simulink model "Copy_of_calibration_pumps"  (R2026a)
settings: Solver=VariableStepAuto  StopTime=inf
StopFcn:
  | Q = out.Q;Q = out.Q;
  | 
  | folder = 'calibration_data';
  | 
  | if ~exist(folder, 'dir')
  |     mkdir(folder);
  | end
  | 
  | baseName = 'pump_calibration';
  | fileName = fullfile(folder, baseName + ".mat");
  | 
  | n = 2;
  | 
  | while exist(fileName, 'file')
  |     fileName = fullfile(folder, baseName + "_" + n + ".mat");
  |     n = n + 1;
  | end
  | 
  | save(fileName, 'Q');
  | 
  | fprintf('Calibration saved to: %s\n', fileName);
values from neighbouring files (symbols this model uses):
  coefficients = [20.111978783 20.2762923351 20.4770477048]    [sensor_calibration.mat]
settings Model: Creator=user  LastModifiedBy=user

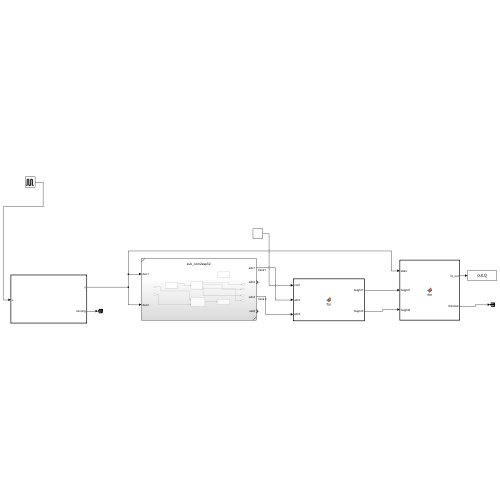
[thumbnail: Simulink's stored preview of the top-level diagram]
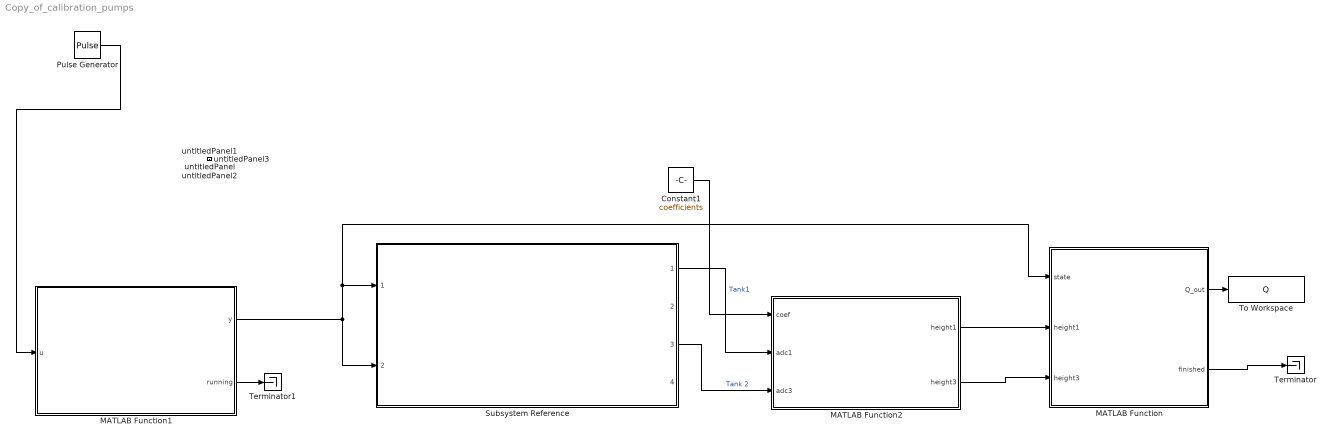
== system Copy_of_calibration_pumps ==
  Constant1 : Constant  Value=coefficients
  MATLAB Function : MATLAB Function  TreatAsAtomicUnit=on
  MATLAB Function1 : MATLAB Function  TreatAsAtomicUnit=on
  MATLAB Function2 : MATLAB Function  TreatAsAtomicUnit=on
  Pulse Generator : DiscretePulseGenerator  PulseType=Time based  Period=12  PulseWidth=20
  Subsystem Reference : Subsystem  ReferencedSubsystem=sub_com2esp32
  Terminator : Terminator
  Terminator1 : Terminator
  To Workspace : ToWorkspace  VariableName=Q  SampleTime=-1
      settings: MaxDataPoints=1
  untitledPanel : Subsystem  Tag=HiddenForWebPanel  IsWebBlockPanel=on
  untitledPanel1 : Subsystem  Tag=HiddenForWebPanel  IsWebBlockPanel=on
  untitledPanel2 : Subsystem  Tag=HiddenForWebPanel  IsWebBlockPanel=on
  untitledPanel3 : Subsystem  Tag=HiddenForWebPanel  IsWebBlockPanel=on
  wires:
  MATLAB Function/1(Q_out) -> To Workspace/1
  MATLAB Function/2(finished) -> Terminator/1
  MATLAB Function1/1(y) -> MATLAB Function/1(state), Subsystem Reference/1, Subsystem Reference/2
  MATLAB Function1/2(running) -> Terminator1/1
  Pulse Generator/1 -> MATLAB Function1/1(u)
  Subsystem Reference/1 -> MATLAB Function2/2(adc1)  "Tank1"
  Subsystem Reference/3 -> MATLAB Function2/3(adc3)  "Tank 2"
  Constant1/1 -> MATLAB Function2/1(coef)
  MATLAB Function2/1(height1) -> MATLAB Function/2(height1)
  MATLAB Function2/2(height3) -> MATLAB Function/3(height3)

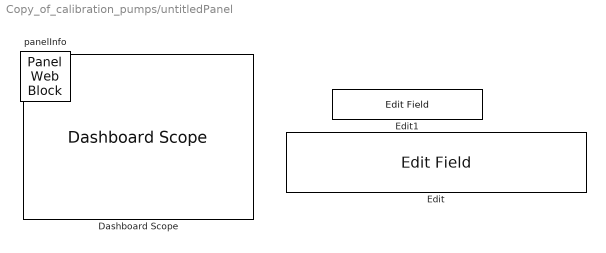
== system Copy_of_calibration_pumps/untitledPanel ==
  Dashboard Scope : DashboardScope  Tag=HiddenForWebPanel  PanelInfo="{\"height\":195,\"left\":22,\"panelId\":\"panelId-0a8f6d05-5e0e-4052-8464-4cdde78ccbfe\",\"top\":22,\"type\":\"panelChild\",\"version\":\"2019b\",\"width\":271,\"zIndex\":1500002}"  FontColor=[0.0, 0.0, 0.0]
  Edit : EditField  Tag=HiddenForWebPanel  PanelInfo="{\"height\":25,\"left\":322,\"panelId\":\"panelId-0a8f6d05-5e0e-4052-8464-4cdde78ccbfe\",\"top\":100,\"type\":\"panelChild\",\"version\":\"2019b\",\"width\":181,\"zIndex\":1500006}"  LabelPosition=Hide  ShowInitialText=on  Alignment=Center
  Edit1 : EditField  Tag=HiddenForWebPanel  PanelInfo="{\"height\":30,\"left\":327,\"panelId\":\"panelId-0a8f6d05-5e0e-4052-8464-4cdde78ccbfe\",\"top\":53,\"type\":\"panelChild\",\"version\":\"2019b\",\"width\":150,\"zIndex\":1500004}"  LabelPosition=Hide  ShowInitialText=on  Alignment=Center
  panelInfo : PanelWebBlock  Tag=HiddenForWebPanel  PanelInfo="{\"compacted\":false,\"height\":362,\"isActiveTab\":false,\"left\":183,\"name\":\"Panel\",\"panelId\":\"panelId-0a8f6d05-5e0e-4052-8464-4cdde78ccbfe\",\"popoutData\":{\"height\":495,\"left\":546,\"maximized\":false,\"top\":827,\"width\":618},\"popoutMode\":\"windowHidden\",\"tabIndex\":0,\"tabbedSetId\":\"tabbedSet4972758365\",\"top\":737,\"type\":\"panel\",\"version\":\"2019b\",\"visible\":false,\"width\":602,\"zIndex\":1500002}"  PanelSnapshot=<binary blob, 20028 chars, not shown>

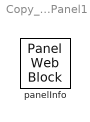
== system Copy_of_calibration_pumps/untitledPanel1 ==
  panelInfo : PanelWebBlock  Tag=HiddenForWebPanel  PanelInfo="{\"compacted\":false,\"height\":362,\"isActiveTab\":true,\"left\":183,\"name\":\"Panel1\",\"panelId\":\"panelId-b2ee2f41-7720-49f1-b51a-3062c351f597\",\"popoutData\":{\"height\":495,\"left\":546,\"maximized\":false,\"top\":827,\"width\":618},\"popoutMode\":\"windowHidden\",\"tabIndex\":1,\"tabbedSetId\":\"tabbedSet4972758365\",\"top\":737,\"type\":\"panel\",\"version\":\"2019b\",\"visible\":true,\"width\":602,\"zIndex\":1500004}"

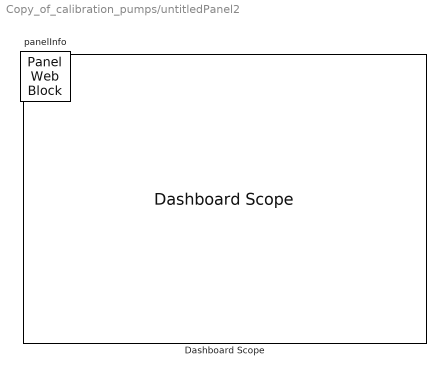
== system Copy_of_calibration_pumps/untitledPanel2 ==
  Dashboard Scope : DashboardScope  Tag=HiddenForWebPanel  PanelInfo="{\"height\":289,\"left\":18,\"panelId\":\"panelId-8ba459e9-7eb9-43d1-9a8b-2b7bff5a2d5c\",\"top\":18,\"type\":\"panelChild\",\"version\":\"2019b\",\"width\":403,\"zIndex\":1500002}"  FontColor=[0.0, 0.0, 0.0]
  panelInfo : PanelWebBlock  Tag=HiddenForWebPanel  PanelInfo="{\"compacted\":false,\"height\":329,\"isActiveTab\":true,\"left\":1320,\"name\":\"Panel2\",\"panelId\":\"panelId-8ba459e9-7eb9-43d1-9a8b-2b7bff5a2d5c\",\"popoutData\":{\"height\":440,\"left\":1683,\"maximized\":false,\"top\":822,\"width\":459},\"popoutMode\":\"windowHidden\",\"tabIndex\":0,\"tabbedSetId\":\"tabbedSet1724704130\",\"top\":710,\"type\":\"panel\",\"version\":\"2019b\",\"visible\":true,\"width\":443,\"zIndex\":1500006}"  PanelSnapshot=<binary blob, 75208 chars, not shown>

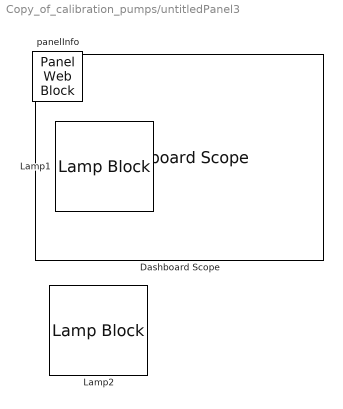
== system Copy_of_calibration_pumps/untitledPanel3 ==
  Dashboard Scope : DashboardScope  Tag=HiddenForWebPanel  PanelInfo="{\"height\":364,\"left\":211,\"panelId\":\"panelId-037cc253-1a0e-430c-bfc3-d197bdfa8fb6\",\"top\":20,\"type\":\"panelChild\",\"version\":\"2019b\",\"width\":531,\"zIndex\":1500002}"  Ymin=0  FontColor=[0.0, 0.0, 0.0]
  Lamp1 : LampBlock  Tag=HiddenForWebPanel  PanelInfo="{\"height\":82,\"left\":28,\"panelId\":\"panelId-037cc253-1a0e-430c-bfc3-d197bdfa8fb6\",\"top\":79,\"type\":\"panelChild\",\"version\":\"2019b\",\"width\":89,\"zIndex\":1500004}"  LabelPosition=Hide  DefaultColor=[192.0, 192.0, 192.0]
  Lamp2 : LampBlock  Tag=HiddenForWebPanel  PanelInfo="{\"height\":82,\"left\":29,\"panelId\":\"panelId-037cc253-1a0e-430c-bfc3-d197bdfa8fb6\",\"top\":226,\"type\":\"panelChild\",\"version\":\"2019b\",\"width\":89,\"zIndex\":1500006}"  LabelPosition=Hide  DefaultColor=[192.0, 192.0, 192.0]
  panelInfo : PanelWebBlock  Tag=HiddenForWebPanel  PanelInfo="{\"compacted\":false,\"height\":411,\"isActiveTab\":true,\"labels\":{\"label0415151059\":{\"deleted\":false,\"left\":29,\"settings\":{\"backgroundColor\":\"rgba(0, 0, 0, 0)\",\"bold\":true,\"font\":\"Arial\",\"fontColor\":\"black\",\"fontSize\":1.09,\"italicized\":false,\"underlined\":false},\"text\":\"Pump\",\"top\":54},\"label6487320007\":{\"deleted\":false,\"left\":27,\"settings\":{\"backgroundColor\":\"rgba(0, 0, 0, 0)\",\"bold\":true,\"font\":\"Arial\",\"fontColor\":\"black\",\"fontSize\":1,\"italicized\":false,\"underlined\":false},\"text\":\"Calibration finished\",\"top\":201}},\"left\":1544,\"name\":\"Panel3\",\"panelId\":\"panelId-037cc253-1a0e-430c-bfc3-d197bdfa8fb6\",\"tabIndex\":0,\"tabbedSetId\":\"tabbedSet3591606152\",\"top\":209,\"type\":\"panel\",\"version\":\"2019b\",\"visible\":true,\"width\":760,\"zIndex\":1500008}"  PanelSnapshot=<binary blob, 44244 chars, not shown>

== matlab function Copy_of_calibration_pumps/MATLAB Function ==
  data: state input; Q_out output; finished output; height1 input; height3 input
function [Q_out, finished] = fcn(state, height1, height3)

persistent sensor_low prev_state Q counter

if isempty(sensor_low)

    sensor_low = zeros(2,1);
    prev_state = 255;
    counter = 0;

    Q = zeros(2,9);

end

A = 154;
dt = 12 * 0.8;

finished = 0;

sensor_now = [height1; height3] * A;

if state ~= 255 && prev_state == 255

    counter = counter + 1;

    if counter <= 8
        sensor_low = sensor_now;
    end

end

if state == 255 && prev_state ~= 255

    if counter >= 1 && counter <= 8

        sensor_high = sensor_now;

        Q(:,counter+1) = ...
            (sensor_high - sensor_low) / dt;

    end

end

if counter >= 8 && state == 255
    finished = 1;
end

prev_state = state;

Q_out = Q;

end

== matlab function Copy_of_calibration_pumps/MATLAB Function1 ==
  data: u input; y output; running output
function [y,running] = fcn(u)
persistent counter2 prev_u

if isempty(counter2) && isempty(prev_u)
    counter2 =0; 
    prev_u =0; 
end
running = 1;

if u ==1 && prev_u ==0
    counter2 = counter2 +1;
end
if u ==0
    s = 0.125 * counter2; 
    if s <= 1
        y = 255 * (1-s);
        running =0;
    else 
        y = 255; 
    end
else
    y = 255; 
end

prev_u = u;

== matlab function Copy_of_calibration_pumps/MATLAB Function2 ==
  data: coef input; height1 output; adc1 input; adc3 input; height3 output
function [height1, height3] = fcn(coef, adc1, adc3)

height1 = ((coef(1,1) * adc1 + coef(1,2)) * adc1 ...
          + coef(1,3)) * adc1 + coef(1,4);

height3 = ((coef(2,1) * adc3 + coef(2,2)) * adc3 ...
          + coef(2,3)) * adc3 + coef(2,4);

end
